simulink model "verify_Collector_1xN_mdl"  (R2018b)
settings: Solver=ode45  StartTime=0  StopTime=24*3600  MaxStep=600  RelTol=1e-3  EnableMultiTasking=on
InitFcn:
  | load('DE_TRY2010_13_averageYear')
libraries: carnot x4
settings Model: Creator=drhf  LastModifiedBy=drhf
settings DataIOCC: SaveFormat=Array  SignalLoggingSaveFormat=ModelDataLogs
settings OptimizationCC: ExpressionDepthLimit=2147483647  LifeSpan=inf
settings DebuggingCC: UnderspecifiedInitializationDetection=Classic  MergeDetectMultiDrivingBlocksExec=none  SolverPrmCheckMsg=warning  FcnCallInpInsideContextMsg=warning  StateNameClashWarn=warning  SFUnexpectedBacktrackingDiag=warning  SFNoUnconditionalDefaultTransitionDiag=warning  SFExecutionAtInitializationDiag=none
settings HardwareCC: ProdBitPerPointer=32  ProdBitPerSizeT=32  ProdBitPerPtrDiffT=32  ProdLargestAtomicFloat=None  ProdIntDivRoundTo=Undefined  ProdEndianess=Unspecified  ProdWordSize=32  ProdHWDeviceType=32-bit Generic
settings ModelReferenceCC: PropagateSignalLabelsOutOfModel=off
settings SFSimCC: SimUseLocalCustomCode=off
settings RTWCC: RTWUseLocalCustomCode=off
settings CodeAppCC: StateflowObjectComments=on
settings GRTTargetCC: TargetLangStandard=C89/C90 (ANSI)  GeneratePreprocessorConditionals=Disable all  CombineOutputUpdateFcns=off  GRTInterface=on
settings ConfigComp: CovMetricSettings=dw  CovHtmlReporting=on  CovSaveCumulativeToWorkspaceVar=on  CovSaveSingleToWorkspaceVar=on  CovExternalEMLEnable=off

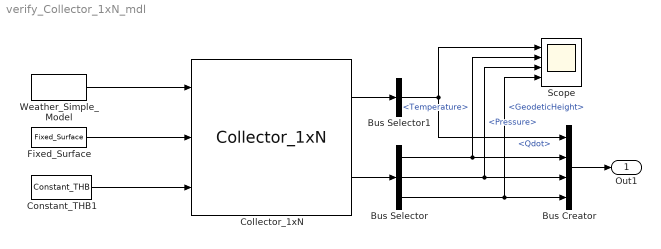
== system verify_Collector_1xN_mdl ==
  Bus Creator : BusCreator  Inputs=4
  Bus Selector : BusSelector  OutputSignals=Temperature,Pressure,GeodeticHeight
  Bus Selector1 : BusSelector  OutputSignals=Qdot
  Collector_1xN : carnot/Source/Solar_Thermal/Collector_1xN  acol=2.3  len=2  eta0=0.8  u1=3.5  u2=0.02  u3=0  uwind=0  c_col=1e4  lin=10  qua=10  tini=20  nodes=5
      settings: SourceProductName=Carnot
  Constant_THB1 : carnot/Source/Simple/Constant_THB  t=40  mdot=100/3600  p=1e5  mID=Full Pressure Drop with Static Height  fluid=Water  mix=0  mix2=0  mix3=0  dia=0.02  hgt=0
      settings: SourceProductName=Carnot
  Fixed_Surface : carnot/Weather/Fixed_Surface  colangle=30  colazi=0  colrot=0
      settings: SourceProductName=Carnot
  Scope : Scope  NumInputPorts=4
  Weather_Simple_Model : carnot/Weather/Weather_Simple_Model  Ibn=900  Idg=100  tamb=5  deltaTsky=-6  rh=50  precip="10e-3/24/3600           % 10 mm in 24 h"  cloud=0.125  p=1013e2  vw=1  wdir=270  lat=60  colangle=0  colazi=0  colrot=0
      settings: SourceProductName=Carnot
  Out1 : Outport
  wires:
  Bus Creator/1 -> Out1/1
  Collector_1xN/2 -> Bus Selector/1
  Bus Selector/1 -> Scope/2, Bus Creator/2  "<Temperature>"
  Bus Selector/2 -> Scope/3, Bus Creator/3  "<Pressure>"
  Weather_Simple_Model/1 -> Collector_1xN/1
  Constant_THB1/1 -> Collector_1xN/3
  Fixed_Surface/1 -> Collector_1xN/2
  Collector_1xN/1 -> Bus Selector1/1
  Bus Selector1/1 -> Bus Creator/1, Scope/1  "<Qdot>"
  Bus Selector/3 -> Scope/4, Bus Creator/4  "<GeodeticHeight>"
